simulink model "zad8"  (R2018a)
settings: Solver=VariableStepAuto  StartTime=0.0  StopTime=1000  RelTol=1e-3
values from neighbouring files (symbols this model uses):
  alfa1 = 0.15    [MODI_Projekt1.m]
  alfa2 = -0.16    [MODI_Projekt1.m]
  alfa3 = 0.25    [MODI_Projekt1.m]
  alfa4 = 0.43    [MODI_Projekt1.m]
  K = 2    [MODI_Projekt1.m]
  T = 1    [MODI_Projekt1.m]
  T1 = 9    [MODI_Projekt1.m]
  T2 = 6    [MODI_Projekt1.m]
  u_p = 0.5    [MODI_Projekt1.m]
  x1_p = 0    [MODI_Projekt1.m]
  x2_p = 0    [MODI_Projekt1.m]
settings Model: Creator=gajee  LastModifiedBy=gajee

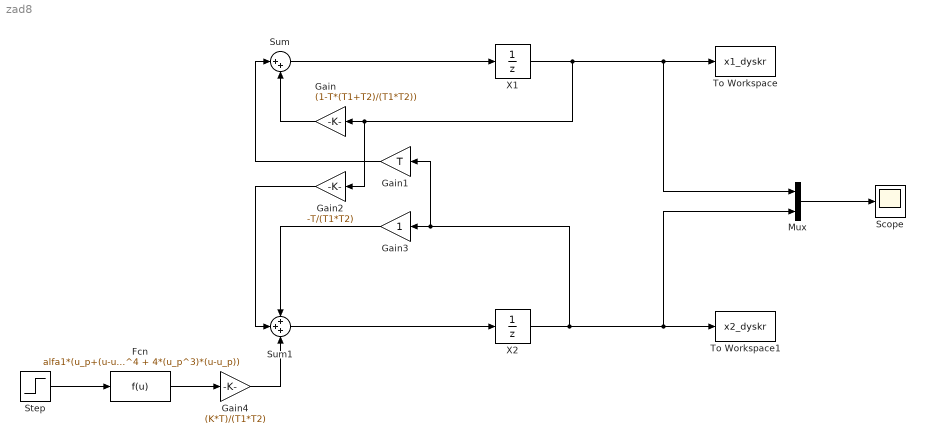
== system zad8 ==
  Fcn : Fcn  Expr=alfa1*(u_p+(u-u_p)) + alfa2*(u_p^2 + 2*u_p*(u-u_p)) +alfa3*(u_p^3 + 3*(u_p^2)*(u-u_p))+alfa4 * (u_p^4 + 4*(u_p^3)*(u-u_p))
  Gain : Gain  Gain=(1-T*(T1+T2)/(T1*T2))
  Gain1 : Gain  Gain=T
  Gain2 : Gain  Gain=-T/(T1*T2)
  Gain3 : Gain
  Gain4 : Gain  Gain=(K*T)/(T1*T2)
  Mux : Mux  Inputs=2
  Scope : Scope
  Step : Step  Before=u_p  After=u  SampleTime=T
  Sum : Sum  Inputs=|++
  Sum1 : Sum  Inputs=+++
  To Workspace : ToWorkspace  VariableName=x1_dyskr  SaveFormat=Structure With Time  SampleTime=-1
  To Workspace1 : ToWorkspace  VariableName=x2_dyskr  SaveFormat=Structure With Time  SampleTime=-1
  "X1 " : UnitDelay  InitialCondition=x1_p  SampleTime=T
  X2 : UnitDelay  InitialCondition=x2_p  SampleTime=T
  wires:
  "X1 "/1 -> Gain2/1, Gain/1, To Workspace/1, Mux/1
  X2/1 -> Gain1/1, Gain3/1, To Workspace1/1, Mux/2
  Gain1/1 -> Sum/1
  Gain/1 -> Sum/2
  Gain2/1 -> Sum1/2
  Gain3/1 -> Sum1/1
  Mux/1 -> Scope/1
  Sum/1 -> "X1 "/1
  Sum1/1 -> X2/1
  Step/1 -> Fcn/1
  Fcn/1 -> Gain4/1
  Gain4/1 -> Sum1/3
